simulink model "BPSK_1"  (R2020a)
settings: Solver=ode45  StartTime=0.0  StopTime=10  RelTol=1e-3  EnableMultiTasking=on
undefined symbols (not defined in the file or in its folder): clock
libraries: simulink_extras x2, commutil2 x2, commchan3 x1, commrandsrc2 x1, simulink x1, commsink2 x1, commfilt2 x1, dspsigops x1
settings Model: Creator=CESAR  LastModifiedBy=L00493460
settings DataIOCC: LimitDataPoints=on  SaveFormat=Array  SignalLoggingSaveFormat=ModelDataLogs  ReturnWorkspaceOutputs=off
settings OptimizationCC: ExpressionDepthLimit=2147483647  LifeSpan=inf
settings DebuggingCC: UnderspecifiedInitializationDetection=Classic  MergeDetectMultiDrivingBlocksExec=none  SolverPrmCheckMsg=warning  FcnCallInpInsideContextMsg=warning  StateNameClashWarn=warning  SFUnexpectedBacktrackingDiag=warning  SFNoUnconditionalDefaultTransitionDiag=warning  SFExecutionAtInitializationDiag=none  ArithmeticOperatorsInVariantConditions=warning
settings HardwareCC: ProdBitPerPointer=32  ProdBitPerSizeT=32  ProdBitPerPtrDiffT=32  ProdLargestAtomicFloat=None  ProdIntDivRoundTo=Undefined  ProdEndianess=Unspecified  ProdWordSize=32  ProdHWDeviceType=32-bit Generic
settings ModelReferenceCC: PropagateSignalLabelsOutOfModel=off
settings SFSimCC: SimUseLocalCustomCode=off  CustomCodeUndefinedFunction=UseInterfaceOnly
settings RTWCC: RTWUseLocalCustomCode=off
settings CodeAppCC: StateflowObjectComments=on
settings GRTTargetCC: TargetLangStandard=C89/C90 (ANSI)  CombineOutputUpdateFcns=off  GRTInterface=on
settings ConfigComp: CovMetricSettings=dw  CovHtmlReporting=on  CovSaveCumulativeToWorkspaceVar=on  CovSaveSingleToWorkspaceVar=on  CovExternalEMLEnable=off  CovSFcnEnable=off

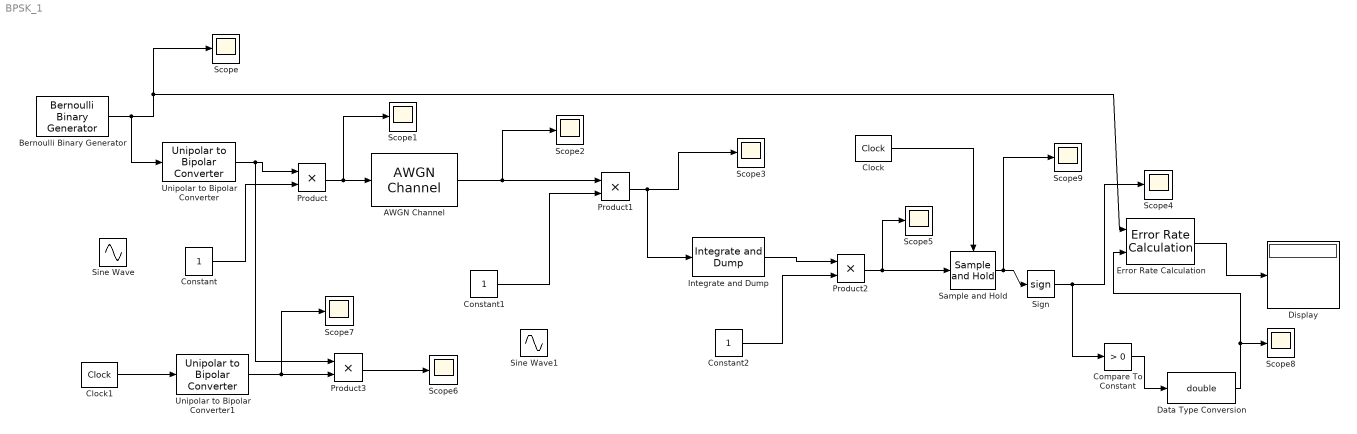
== system BPSK_1 ==
  AWGN Channel : commchan3/AWGN Channel  InputProcessing=Columns as channels (frame based)  seed=sum(100*clock)  noiseMode="Signal to noise ratio  (Eb/No)"  EbNodB=50  EsNodB=20  SNRdB=10  bitsPerSym=1  Ps=1  Tsym=1  variance=1
  Bernoulli Binary Generator : commrandsrc2/Bernoulli Binary Generator  P=0.5  seed=sum(100*clock)  Ts=1  frameBased=off  sampPerFrame=1  orient=off  outDataType=double
      settings: SourceProductBaseCode=CM
  Clock : simulink_extras/Flip Flops/Clock  period=0.99999
  Clock1 : simulink_extras/Flip Flops/Clock  period=1
  Compare To Constant : simulink/Logic and Bit Operations/Compare To Constant  relop=>  const=0  OutDataTypeStr=uint8  ZeroCross=off
  Constant : Constant  SampleTime=1/1000
  Constant1 : Constant
  Constant2 : Constant
  Data Type Conversion : DataTypeConversion  OutDataTypeStr=double  RndMeth=Ceiling  SampleTime=1  SaturateOnIntegerOverflow=on
  Display : Display
  Error Rate Calculation : commsink2/Error Rate Calculation  N=1  st_delay=0  cp_mode=Entire frame  subframe=[]  PMode=Port  WsName=ErrorVec  RsMode2=off  stop=off  numErr=100  maxBits=1e6
  Integrate and Dump : commfilt2/Integrate and Dump  obssamples=1000  offsetsamples=0  nodump=on  roundingMode=Floor  overflowMode=off  outputDataTypeStr=Inherit: Same as accumulator  outputLastDataTypeStr=Inherit: Same as accumulator
  Product{,1..3} (4 alike) : Product  RndMeth=Zero
  Sample and Hold : dspsigops/Sample and Hold  trig=Rising edge  initCond=0  latchinput=off
  Scope{,1..9} (10 alike) : Scope
  Sign : Signum
  Sine Wave : Sin  Frequency=2*pi*3  SampleTime=1/1000
  Sine Wave1 : Sin  Frequency=2*pi*3  SampleTime=1/1000
  Unipolar to Bipolar Converter : commutil2/Unipolar to Bipolar Converter  M=2  polarity=Positive  dataType=Inherit via internal rule
  Unipolar to Bipolar Converter1 : commutil2/Unipolar to Bipolar Converter  M=2  polarity=Positive  dataType=Inherit via internal rule
  wires:
  Bernoulli Binary Generator/1 -> Unipolar to Bipolar Converter/1, Scope/1, Error Rate Calculation/1
  Unipolar to Bipolar Converter/1 -> Product3/1, Product/1
  Product/1 -> AWGN Channel/1, Scope1/1
  AWGN Channel/1 -> Scope2/1, Product1/1
  Product1/1 -> Scope3/1, Integrate and Dump/1
  Integrate and Dump/1 -> Product2/1
  Constant2/1 -> Product2/2
  Product2/1 -> Sample and Hold/1, Scope5/1
  Sample and Hold/1 -> Scope9/1, Sign/1
  Sign/1 -> Scope4/1, Compare To Constant/1
  Error Rate Calculation/1 -> Display/1
  Compare To Constant/1 -> Data Type Conversion/1
  Data Type Conversion/1 -> Scope8/1, Error Rate Calculation/2
  Product3/1 -> Scope6/1
  Clock1/1 -> Unipolar to Bipolar Converter1/1
  Unipolar to Bipolar Converter1/1 -> Scope7/1, Product3/2
  Clock/1 -> Sample and Hold/Trigger
  Constant/1 -> Product/2
  Constant1/1 -> Product1/2
